simulink library "PB_Library_Master_Working"  (R2021a)
settings: Solver=VariableStepAuto  StartTime=0.0  StopTime=10.0  RelTol=1e-3
undefined symbols (not defined in the file): A_M, B_M, component_degradation_input, E0_M, f_sw, f_sw_M_aDF, flux_m_aDF, Fsw_M_aDF, insert, K_M, L_M_aDF, L_M_adf, P_Fe_Nom_aDF, Q_M, Q_rr, r_c, r_D, R_M, R_s_aDF, resistance_aDF, S_nom_aDF, SOC_Init_M, TFall_M_aDF, TRise_M_aDF, Trr_M_aDF, u_ce0, u_D0
libraries: $bdroot x76, Lib_Dyn_StateSpace_EMTAT x6, Lib_PF_BusLoadDC_TMATS x3, PB_Library_Master x3, simulink x3, TemperatureBlock x1
(part 4 of 5)

== system PB_Library_Master_Working/Rectifier/IGBT Conduction Losses1 ==
  note: You need to read from graphs:
      |
      | -U_ce0
      | -Rc=dU_ce/dI_c (linear)
      | -U_D0
      | -R_D=dU_D/dI_D (linear)
  I_M : Inport
  PF : Inport  Port=2
  m : Inport  Port=3
  T : Inport  Port=4
  1-D Lookup Table r_c : Lookup_n-D  NumberOfTableDimensions=1  BreakpointsForDimension1=T_M  Table=R_c_M  InternalRulePriority=Speed  RndMeth=Simplest  InputSameDT=on
  1-D Lookup Table u_ce0 : Lookup_n-D  NumberOfTableDimensions=1  BreakpointsForDimension1=T_M  Table=u_ce0_M  InternalRulePriority=Speed  RndMeth=Simplest  InputSameDT=on
  Constant : Constant  Value=1/(2*pi)
  Constant1 : Constant  Value=1/8
  Gain : Gain  Commented=on  Gain=u_ce0
  Gain1 : Gain  Gain=1/8
  Gain2 : Gain  Commented=on  Gain=r_c
  Gain3 : Gain  Gain=1/(3*pi)
  Product{,1..4} (5 alike) : Product
  Square : Math  Operator=square  SignedPower=on  SaturateOnIntegerOverflow=on
  Sum : Sum
  Sum2 : Sum
  Sum3 : Sum
  P_CT : Outport  VectorParamsAs1DForOutWhenUnconnected=off
  wires:
  1-D Lookup Table r_c/1 -> Product4/2
  1-D Lookup Table u_ce0/1 -> Product3/2
  T/1 -> 1-D Lookup Table r_c/1, 1-D Lookup Table u_ce0/1
  Sum3/1 -> Product2/2
  Constant1/1 -> Sum3/2
  Product4/1 -> Product2/1
  Gain3/1 -> Sum3/1
  Square/1 -> Product4/1
  Sum/1 -> Product/1
  Product1/1 -> Gain1/1, Gain3/1
  Gain1/1 -> Sum/2
  m/1 -> Product1/2
  PF/1 -> Product1/1
  Constant/1 -> Sum/1
  Product3/1 -> Square/1, Product/2
  I_M/1 -> Product3/1  "I_M"
  Sum2/1 -> P_CT/1
  Product2/1 -> Sum2/2
  Product/1 -> Sum2/1

== system PB_Library_Master_Working/Rectifier/IGBT Switching Losses1 ==
  note: the aDF must increase E1_M
  I_ce : Inport
  T : Inport  Port=2
  1-D Lookup Table E0 : Lookup_n-D  NumberOfTableDimensions=1  BreakpointsForDimension1=T_M  Table=E0_M  InternalRulePriority=Speed  RndMeth=Simplest  InputSameDT=on
  1-D Lookup Table E1 : Lookup_n-D  NumberOfTableDimensions=1  BreakpointsForDimension1=T_M  Table=E1_M  InternalRulePriority=Speed  RndMeth=Simplest  InputSameDT=on
  Add : Sum
  Constant : Constant  Value=f_sw_M
  Constant1 : Constant  Value=[insert f_sw_M_aDF]
  Divide : Product  Inputs=*/
  Product : Product
  Product1 : Product
  P_ST : Outport  VectorParamsAs1DForOutWhenUnconnected=off
  wires:
  Product/1 -> P_ST/1
  Add/1 -> Product/1
  I_ce/1 -> Product1/1
  1-D Lookup Table E0/1 -> Add/1
  Product1/1 -> Add/2
  T/1 -> 1-D Lookup Table E0/1, 1-D Lookup Table E1/1
  1-D Lookup Table E1/1 -> Product1/2
  Constant/1 -> Divide/1
  Divide/1 -> Product/2
  Constant1/1 -> Divide/2

== system PB_Library_Master_Working/Rectifier/I_Ripple1 ==
  V_batt : Inport
  "V_M " : Inport  Port=2
  Constant : Constant  Value=L_s_M
  Constant1 : Constant  Value=[insert f_sw_M_aDF]
  Divide : Product  Inputs=*/
  Divide1 : Product  Inputs=*/
  Gain : Gain  Gain=sqrt(2)
  Gain1 : Gain  Gain=2
  Gain2 : Gain  Gain=f_sw_M
  Product : Product
  Product1 : Product
  Subtract : Sum  Inputs=+-
  I_Rip : Outport  VectorParamsAs1DForOutWhenUnconnected=off
  wires:
  Divide/1 -> I_Rip/1
  Product1/1 -> Gain2/1
  Gain1/1 -> Product1/2
  Constant/1 -> Gain1/1
  Product/1 -> Divide/1
  Subtract/1 -> Product/1
  V_batt/1 -> Product1/1, Subtract/1
  Gain/1 -> Subtract/2
  "V_M "/1 -> Gain/1, Product/2
  Gain2/1 -> Divide1/1
  Constant1/1 -> Divide1/2
  Divide1/1 -> Divide/2

== system PB_Library_Master_Working/Rectifier/P_out_gen ==
  I (RMS) : Inport
  V_s (RMS) : Inport  Port=2
  PF : Inport  Port=3
  Gain : Gain  Gain=sqrt(3)
  Product : Product  Inputs=3
  P_out_gen : Outport  VectorParamsAs1DForOutWhenUnconnected=off
  wires:
  Product/1 -> Gain/1
  Gain/1 -> P_out_gen/1
  V_s (RMS)/1 -> Product/1
  PF/1 -> Product/3
  I (RMS)/1 -> Product/2

== system PB_Library_Master_Working/Rectifier/mVal ==
  V_s : Inport
  V_batt : Inport  Port=2
  Divide : Product  Inputs=*/
  Gain : Gain  Gain=sqrt(2)
  m : Outport  VectorParamsAs1DForOutWhenUnconnected=off
  wires:
  V_batt/1 -> Divide/2
  Gain/1 -> Divide/1
  V_s/1 -> Gain/1
  Divide/1 -> m/1

== system PB_Library_Master_Working/Boost Converter/DC - DC Converter/ Dynamic State ==
  note: On Cycle
  note: Off Cycle
  x : Inport
  u : Inport  Port=2
  d : Inport  Port=3
  Action Port : ActionPort
  Constant : Constant
  Product{,1..3} (4 alike) : Product
  "State Space Model A1, B1, C1, D1" : Lib_Dyn_StateSpace_EMTAT/State Space Model  A_M=[0, 0; 0, -(Ron_M+RL_M)/L_M]  B_M=[0, -1/C_M; 1/L_M, 0]  C_M="[1,  0]"  D_M=[0, RC_M]
  "State Space Model A2, B2, C2, D2" : Subsystem  mask(State Space Model){A_M=[0, 1/C_M; -1/L_M, -(Ron_M+RC_M+RL_M)/L_M], B_M=[0, -1/C_M; 1/L_M, RC_M/L_M], C_M=[1,  RC_M], D_M=[0, -RC_M]}
      mask prompts: A_M "A_M - "A" Matrix"; B_M "B_M - "B" Matrix"; C_M "C_M - "C" Matrix"; D_M "D_M - "D" Matrix"
      mask help:
      | This block represents a state space model that can be placed within an interative subsytem (i.e. the Newton-Raphson solver).
      | The states, x, and inputs, u must be fed into the block. The outputs, y, and state derivatives, x_dot are computed
      | via the standard state space equations. Note that the integrator that computes the states by integrating
      | the state derivatives should be placed outside of the iterative subsystem so that multiple integration steps do not
      | occur per each timestep.
      |
      | Initial conditions must be specified in the integrator blocks, and ABCD matrices specified as block mask parameters.
      mask Display:
      | fprintf('x_dot = Ax+Bu\ny = Cx+Du')
      | port_label('input',1,'x')
      | port_label('input',2,'u')
      | port_label('output',1,'x_dot')
      | port_label('output',2,'y')
  Sum : Sum  Inputs=++|
  Sum1 : Sum  Inputs=++|
  Sum2 : Sum  Inputs=+-
  xdot : Outport  VectorParamsAs1DForOutWhenUnconnected=off
  VB : Outport  Port=2  VectorParamsAs1DForOutWhenUnconnected=off
  wires:
  "State Space Model A1, B1, C1, D1"/1 -> Product/1
  d/1 -> [d]
  Sum2/1 -> Product2/2, Product3/2
  Constant/1 -> Sum2/1
  [x] -> "State Space Model A1, B1, C1, D1"/1
  "State Space Model A1, B1, C1, D1"/2 -> Product1/1
  [u] -> "State Space Model A1, B1, C1, D1"/2
  [d] -> Product1/2, Product/2
  [d] -> Sum2/2
  u/1 -> [u]
  [x] -> "State Space Model A2, B2, C2, D2"/1(x)
  [u] -> "State Space Model A2, B2, C2, D2"/2(u)
  Product3/1 -> Sum1/2
  "State Space Model A2, B2, C2, D2"/2(y) -> Product3/1
  "State Space Model A2, B2, C2, D2"/1(x_dot) -> Product2/1
  Product2/1 -> Sum/2
  x/1 -> [x]
  Product1/1 -> Sum1/1
  Product/1 -> Sum/1
  Sum1/1 -> VB/1  "VB"
  Sum/1 -> xdot/1  "xdot"

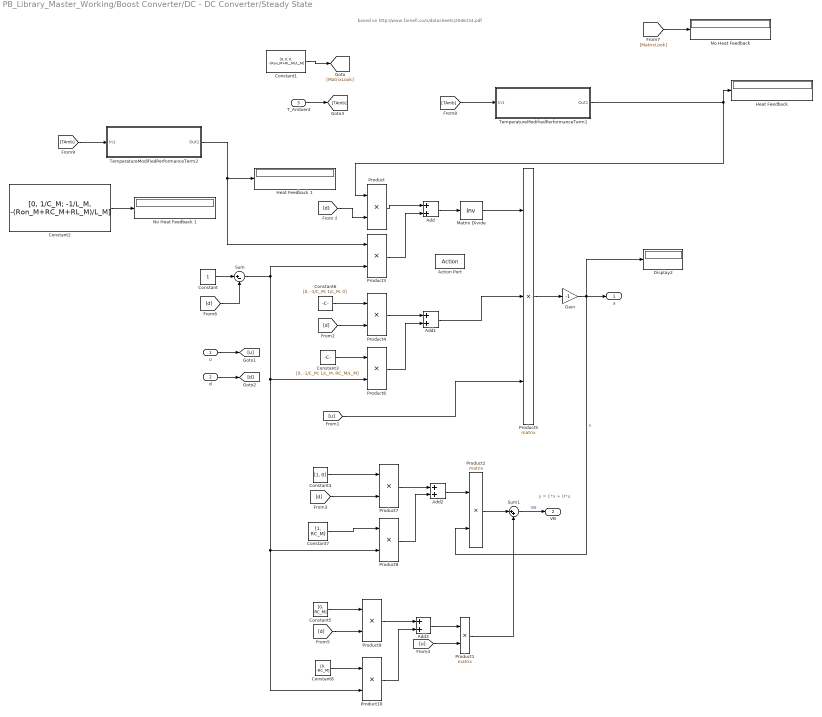
== system PB_Library_Master_Working/Boost Converter/DC - DC Converter/Steady State ==
  note: based on http://www.farnell.com/datasheets/2046154.pdf
  note: d
  note: y = C*x + D*u
  u : Inport
  d : Inport  Port=2
  "T_Ambient " : Inport  Port=3
  Action Port : ActionPort
  Add{,1..3} (4 alike) : Sum
  Constant : Constant
  Constant1 : Constant  Value=[0, 0; 0, -(Ron_M+RL_M)/L_M]  VectorParams1D=off
  Constant2 : Constant  Value=[0, 1/C_M; -1/L_M, -(Ron_M+RC_M+RL_M)/L_M]  VectorParams1D=off
  Constant3 : Constant  Value=[0, -1/C_M; 1/L_M, RC_M/L_M]  VectorParams1D=off
  Constant4 : Constant  Value=[1, 0]  VectorParams1D=off
  Constant5 : Constant  Value=[0, RC_M]  VectorParams1D=off
  Constant6 : Constant  Value=[0, -1/C_M; 1/L_M, 0]  VectorParams1D=off
  Constant7 : Constant  Value=[1, RC_M]  VectorParams1D=off
  Constant8 : Constant  Value=[0, -RC_M]  VectorParams1D=off
  Display2 : Display
  Gain : Gain  Gain=-1
  "Heat Feedback " : Display
  Heat Feedback 1 : Display
  Matrix Divide : Product  Inputs=/  Multiplication=Matrix(*)
  "No Heat Feedback " : Display
  No Heat Feedback 1 : Display
  Product{,3..4,6..10} (8 alike) : Product
  Product1 : Product  Multiplication=Matrix(*)
  Product2 : Product  Multiplication=Matrix(*)
  Product5 : Product  Inputs=3  Multiplication=Matrix(*)
  Sum : Sum  Inputs=|+-
  Sum1 : Sum  Inputs=|++
  "TemperatureModifiedPerformanceTerm1 " : Subsystem
  "TemperatureModifiedPerformanceTerm2 " : Subsystem
  x : Outport  VectorParamsAs1DForOutWhenUnconnected=off
  VB : Outport  Port=2  VectorParamsAs1DForOutWhenUnconnected=off
  wires:
  Constant2/1 -> No Heat Feedback 1/1
  [TAmb] -> "TemperatureModifiedPerformanceTerm2 "/1(In1)
  [TAmb] -> "TemperatureModifiedPerformanceTerm1 "/1(In1)
  "T_Ambient "/1 -> [TAmb]
  "TemperatureModifiedPerformanceTerm2 "/1(Out1) -> Heat Feedback 1/1, Product3/1
  "TemperatureModifiedPerformanceTerm1 "/1(Out1) -> Product/1, "Heat Feedback "/1
  [d] -> Product/2
  [MatrixLook] -> "No Heat Feedback "/1
  Constant8/1 -> Product10/1
  Product6/1 -> Add1/2
  Add/1 -> Matrix Divide/1
  Constant7/1 -> Product8/1
  [d] -> Product7/2
  Add1/1 -> Product5/2
  Product8/1 -> Add2/2
  Product10/1 -> Add3/2
  Constant5/1 -> Product9/1
  [d] -> Sum/2
  Product1/1 -> Sum1/2
  Product5/1 -> Gain/1
  Sum/1 -> Product10/2, Product8/2, Product6/2, Product3/2
  Add3/1 -> Product1/1
  Constant/1 -> Sum/1
  Constant6/1 -> Product4/1
  [u] -> Product5/3
  [d] -> Product4/2
  Gain/1 -> x/1, Display2/1, Product2/2  "x"
  Constant4/1 -> Product7/1
  u/1 -> [u]
  Product2/1 -> Sum1/1
  d/1 -> [d]
  Product7/1 -> Add2/1
  Sum1/1 -> VB/1  "VB"
  Constant1/1 -> [MatrixLook]
  Product4/1 -> Add1/1
  [d] -> Product9/2
  Product/1 -> Add/1
  Constant3/1 -> Product6/1
  Product3/1 -> Add/2
  Matrix Divide/1 -> Product5/1
  Product9/1 -> Add3/1
  Add2/1 -> Product2/1
  [u] -> Product1/2

== system PB_Library_Master_Working/Boost Converter/Power Loss /VGateTempModified ==
  note: normalized to 25°C
  VGate : Inport
  TAmb : Inport  Port=2
  Add1 : Sum
  Constant7 : Constant  Value=25
  Multiply1 : Product
  Subtract : Sum  Inputs=+-
  "V DS temp coefficient " : Constant  Value=.64
  VGateMod : Outport  VectorParamsAs1DForOutWhenUnconnected=off
  wires:
  Add1/1 -> VGateMod/1
  "V DS temp coefficient "/1 -> Multiply1/2
  Subtract/1 -> Multiply1/1
  TAmb/1 -> Subtract/1
  VGate/1 -> Add1/1
  Constant7/1 -> Subtract/2
  Multiply1/1 -> Add1/2

== system PB_Library_Master_Working/Boost Converter Analytic/DC - DC Converter/ Dynamic State ==
  note: On Cycle
  note: Off Cycle
  note: the aDF must decrease L_M
  note: the aDF must decrease L_M
  x : Inport
  u : Inport  Port=2
  d : Inport  Port=3
  Action Port : ActionPort
  Constant : Constant
  Product{,1..3} (4 alike) : Product
  "State Space Model A1, B1, C1, D1" : Lib_Dyn_StateSpace_EMTAT/State Space Model  A_M=[0, 0; 0, -(Ron_M+RL_M)/L_M]  B_M=[0, -1/C_M; 1/L_M, 0]  C_M="[1,  0]"  D_M=[0, RC_M]
  "State Space Model A2, B2, C2, D2" : Subsystem  mask(State Space Model){A_M=[0, 1/C_M; -1/L_M, -(Ron_M+RC_M+RL_M)/L_M], B_M=[0, -1/C_M; 1/L_M, RC_M/L_M], C_M=[1,  RC_M], D_M=[0, -RC_M]}
      mask prompts: A_M "A_M - "A" Matrix"; B_M "B_M - "B" Matrix"; C_M "C_M - "C" Matrix"; D_M "D_M - "D" Matrix"
      mask help:
      | This block represents a state space model that can be placed within an interative subsytem (i.e. the Newton-Raphson solver).
      | The states, x, and inputs, u must be fed into the block. The outputs, y, and state derivatives, x_dot are computed
      | via the standard state space equations. Note that the integrator that computes the states by integrating
      | the state derivatives should be placed outside of the iterative subsystem so that multiple integration steps do not
      | occur per each timestep.
      |
      | Initial conditions must be specified in the integrator blocks, and ABCD matrices specified as block mask parameters.
      mask Display:
      | fprintf('x_dot = Ax+Bu\ny = Cx+Du')
      | port_label('input',1,'x')
      | port_label('input',2,'u')
      | port_label('output',1,'x_dot')
      | port_label('output',2,'y')
  Sum : Sum  Inputs=++|
  Sum1 : Sum  Inputs=++|
  Sum2 : Sum  Inputs=+-
  xdot : Outport  VectorParamsAs1DForOutWhenUnconnected=off
  VB : Outport  Port=2  VectorParamsAs1DForOutWhenUnconnected=off
  wires:
  "State Space Model A1, B1, C1, D1"/1 -> Product/1
  d/1 -> [d]
  Sum2/1 -> Product2/2, Product3/2
  Constant/1 -> Sum2/1
  [x] -> "State Space Model A1, B1, C1, D1"/1
  "State Space Model A1, B1, C1, D1"/2 -> Product1/1
  [u] -> "State Space Model A1, B1, C1, D1"/2
  [d] -> Product1/2, Product/2
  [d] -> Sum2/2
  u/1 -> [u]
  [x] -> "State Space Model A2, B2, C2, D2"/1(x)
  [u] -> "State Space Model A2, B2, C2, D2"/2(u)
  Product3/1 -> Sum1/2
  "State Space Model A2, B2, C2, D2"/2(y) -> Product3/1
  "State Space Model A2, B2, C2, D2"/1(x_dot) -> Product2/1
  Product2/1 -> Sum/2
  x/1 -> [x]
  Product1/1 -> Sum1/1
  Product/1 -> Sum/1
  Sum1/1 -> VB/1  "VB"
  Sum/1 -> xdot/1  "xdot"

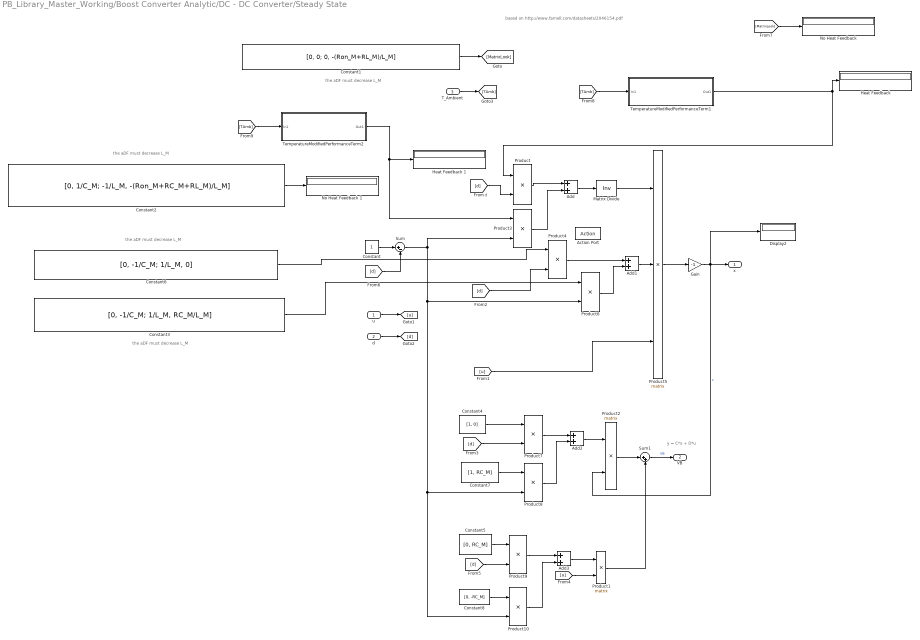
== system PB_Library_Master_Working/Boost Converter Analytic/DC - DC Converter/Steady State ==
  note: the aDF must decrease L_M
  note: based on http://www.farnell.com/datasheets/2046154.pdf
  note: d
  note: y = C*x + D*u
  note: the aDF must decrease L_M
  note: the aDF must decrease L_M
  note: the aDF must decrease L_M
  u : Inport
  d : Inport  Port=2
  "T_Ambient " : Inport  Port=3
  Action Port : ActionPort
  Add{,1..3} (4 alike) : Sum
  Constant : Constant
  Constant1 : Constant  Value=[0, 0; 0, -(Ron_M+RL_M)/L_M]  VectorParams1D=off
  Constant2 : Constant  Value=[0, 1/C_M; -1/L_M, -(Ron_M+RC_M+RL_M)/L_M]  VectorParams1D=off
  Constant3 : Constant  Value=[0, -1/C_M; 1/L_M, RC_M/L_M]  VectorParams1D=off
  Constant4 : Constant  Value=[1, 0]  VectorParams1D=off
  Constant5 : Constant  Value=[0, RC_M]  VectorParams1D=off
  Constant6 : Constant  Value=[0, -1/C_M; 1/L_M, 0]  VectorParams1D=off
  Constant7 : Constant  Value=[1, RC_M]  VectorParams1D=off
  Constant8 : Constant  Value=[0, -RC_M]  VectorParams1D=off
  Display2 : Display
  Gain : Gain  Gain=-1
  "Heat Feedback " : Display
  Heat Feedback 1 : Display
  Matrix Divide : Product  Inputs=/  Multiplication=Matrix(*)
  "No Heat Feedback " : Display
  No Heat Feedback 1 : Display
  Product{,3..4,6..10} (8 alike) : Product
  Product1 : Product  Multiplication=Matrix(*)
  Product2 : Product  Multiplication=Matrix(*)
  Product5 : Product  Inputs=3  Multiplication=Matrix(*)
  Sum : Sum  Inputs=|+-
  Sum1 : Sum  Inputs=|++
  "TemperatureModifiedPerformanceTerm1 " : Subsystem
  "TemperatureModifiedPerformanceTerm2 " : Subsystem
  x : Outport  VectorParamsAs1DForOutWhenUnconnected=off
  VB : Outport  Port=2  VectorParamsAs1DForOutWhenUnconnected=off
  wires:
  Constant2/1 -> No Heat Feedback 1/1
  [TAmb] -> "TemperatureModifiedPerformanceTerm2 "/1(In1)
  [TAmb] -> "TemperatureModifiedPerformanceTerm1 "/1(In1)
  "T_Ambient "/1 -> [TAmb]
  "TemperatureModifiedPerformanceTerm2 "/1(Out1) -> Heat Feedback 1/1, Product3/1
  "TemperatureModifiedPerformanceTerm1 "/1(Out1) -> Product/1, "Heat Feedback "/1
  [d] -> Product/2
  [MatrixLook] -> "No Heat Feedback "/1
  Constant8/1 -> Product10/1
  Product6/1 -> Add1/2
  Add/1 -> Matrix Divide/1
  Constant7/1 -> Product8/1
  [d] -> Product7/2
  Add1/1 -> Product5/2
  Product8/1 -> Add2/2
  Product10/1 -> Add3/2
  Constant5/1 -> Product9/1
  [d] -> Sum/2
  Product1/1 -> Sum1/2
  Product5/1 -> Gain/1
  Sum/1 -> Product10/2, Product8/2, Product6/2, Product3/2
  Add3/1 -> Product1/1
  Constant/1 -> Sum/1
  Constant6/1 -> Product4/1
  [u] -> Product5/3
  [d] -> Product4/2
  Gain/1 -> x/1, Display2/1, Product2/2  "x"
  Constant4/1 -> Product7/1
  u/1 -> [u]
  Product2/1 -> Sum1/1
  d/1 -> [d]
  Product7/1 -> Add2/1
  Sum1/1 -> VB/1  "VB"
  Constant1/1 -> [MatrixLook]
  Product4/1 -> Add1/1
  [d] -> Product9/2
  Product/1 -> Add/1
  Constant3/1 -> Product6/1
  Product3/1 -> Add/2
  Matrix Divide/1 -> Product5/1
  Product9/1 -> Add3/1
  Add2/1 -> Product2/1
  [u] -> Product1/2

== system PB_Library_Master_Working/Boost Converter Analytic/Power Loss /VGateTempModified ==
  note: normalized to 25°C
  VGate : Inport
  TAmb : Inport  Port=2
  Add1 : Sum
  Constant7 : Constant  Value=25
  Multiply1 : Product
  Subtract : Sum  Inputs=+-
  "V DS temp coefficient " : Constant  Value=.64
  VGateMod : Outport  VectorParamsAs1DForOutWhenUnconnected=off
  wires:
  Add1/1 -> VGateMod/1
  "V DS temp coefficient "/1 -> Multiply1/2
  Subtract/1 -> Multiply1/1
  TAmb/1 -> Subtract/1
  VGate/1 -> Add1/1
  Constant7/1 -> Subtract/2
  Multiply1/1 -> Add1/2

== system PB_Library_Master_Working/Buck Converter/DC - DC Converter/ Dynamic State ==
  x : Inport
  u : Inport  Port=2
  d : Inport  Port=3
  Action Port : ActionPort
  Constant : Constant
  Product{,1..3} (4 alike) : Product
  "State Space Model A1, B1, C1, D1" : Lib_Dyn_StateSpace_EMTAT/State Space Model  A_M=[0, 1/C_M; -1/L_M, -(Ron_M+RC_M+RL_M)/L_M]  B_M=[0, -1/C_M; 1/L_M, RC_M/L_M]  C_M="[1,  RC_M]"  D_M=[0, -RC_M]
  "State Space Model A2, B2, C2, D2" : Lib_Dyn_StateSpace_EMTAT/State Space Model  A_M=[0, 1/C_M; -1/L_M, -(Ron_M+RC_M+RL_M)/L_M]  B_M=[0, -1/C_M; 0, RC_M/L_M]  C_M="[1,  RC_M]"  D_M=[0, -RC_M]
  Sum : Sum  Inputs=++|
  Sum1 : Sum  Inputs=++|
  Sum2 : Sum  Inputs=+-
  xdot : Outport  VectorParamsAs1DForOutWhenUnconnected=off
  VB : Outport  Port=2  VectorParamsAs1DForOutWhenUnconnected=off
  wires:
  "State Space Model A1, B1, C1, D1"/1 -> Product/1
  d/1 -> [d]
  Sum2/1 -> Product2/2, Product3/2
  Constant/1 -> Sum2/1
  [x] -> "State Space Model A1, B1, C1, D1"/1
  "State Space Model A1, B1, C1, D1"/2 -> Product1/1
  [u] -> "State Space Model A1, B1, C1, D1"/2
  [d] -> Product1/2, Product/2
  [d] -> Sum2/2
  u/1 -> [u]
  [x] -> "State Space Model A2, B2, C2, D2"/1
  [u] -> "State Space Model A2, B2, C2, D2"/2
  Product3/1 -> Sum1/2
  "State Space Model A2, B2, C2, D2"/2 -> Product3/1
  "State Space Model A2, B2, C2, D2"/1 -> Product2/1
  Product2/1 -> Sum/2
  x/1 -> [x]
  Product1/1 -> Sum1/1
  Product/1 -> Sum/1
  Sum1/1 -> VB/1  "VB"
  Sum/1 -> xdot/1  "xdot"

== system PB_Library_Master_Working/Buck Converter/DC - DC Converter/Steady State ==
  note: d
  note: y = C*x + D*u
  u : Inport
  d : Inport  Port=2
  "T_Ambient " : Inport  Port=3
  Action Port : ActionPort
  Add{,1..3} (4 alike) : Sum
  Constant : Constant
  Constant3 : Constant  Value=[0, -1/C_M; 0, RC_M/L_M]  VectorParams1D=off
  Constant4 : Constant  Value=[1, RC_M]  VectorParams1D=off
  Constant5 : Constant  Value=[0, -RC_M]  VectorParams1D=off
  Constant6 : Constant  Value=[0, -1/C_M; 1/L_M, RC_M]  VectorParams1D=off
  Constant7 : Constant  Value=[1, RC_M]  VectorParams1D=off
  Constant8 : Constant  Value=[0, -RC_M]  VectorParams1D=off
  Gain : Gain  Gain=-1
  Matrix Divide : Product  Inputs=/  Multiplication=Matrix(*)
  Product{,3..4,6..10} (8 alike) : Product
  Product1 : Product  Multiplication=Matrix(*)
  Product2 : Product  Multiplication=Matrix(*)
  Product5 : Product  Inputs=3  Multiplication=Matrix(*)
  Sum : Sum  Inputs=|+-
  Sum1 : Sum  Inputs=|++
  "TemperatureModifiedPerformanceTerm2 " : Subsystem
  x : Outport  VectorParamsAs1DForOutWhenUnconnected=off
  VB : Outport  Port=2  VectorParamsAs1DForOutWhenUnconnected=off
  wires:
  "T_Ambient "/1 -> "TemperatureModifiedPerformanceTerm2 "/1(TAmbient)
  "TemperatureModifiedPerformanceTerm2 "/1(Out1) -> Product3/1, Product/1
  Constant8/1 -> Product10/1
  Product6/1 -> Add1/2
  Add/1 -> Matrix Divide/1
  Constant7/1 -> Product8/1
  [d] -> Product7/2
  Add1/1 -> Product5/2
  Product8/1 -> Add2/2
  Product10/1 -> Add3/2
  [d] -> Product/2
  Constant5/1 -> Product9/1
  [d] -> Sum/2
  Product1/1 -> Sum1/2
  Product5/1 -> Gain/1
  Sum/1 -> Product10/2, Product8/2, Product6/2, Product3/2
  Add3/1 -> Product1/1
  Constant/1 -> Sum/1
  Constant6/1 -> Product4/1
  [u] -> Product5/3
  [d] -> Product4/2
  Gain/1 -> x/1, Product2/2  "x"
  Constant4/1 -> Product7/1
  u/1 -> [u]
  Product2/1 -> Sum1/1
  d/1 -> [d]
  Product7/1 -> Add2/1
  Sum1/1 -> VB/1  "VB"
  Product4/1 -> Add1/1
  [d] -> Product9/2
  Product/1 -> Add/1
  Constant3/1 -> Product6/1
  Product3/1 -> Add/2
  Matrix Divide/1 -> Product5/1
  Product9/1 -> Add3/1
  Add2/1 -> Product2/1
  [u] -> Product1/2

== system PB_Library_Master_Working/Buck Converter/Power Loss /VGateTempModified ==
  note: normalized to 25°C
  "VGate " : Inport
  TAmb : Inport  Port=2
  Add1 : Sum
  Constant7 : Constant  Value=25
  Multiply1 : Product
  Subtract : Sum  Inputs=+-
  "V DS temp coefficient " : Constant  Value=.64
  "VGateMod " : Outport  VectorParamsAs1DForOutWhenUnconnected=off
  wires:
  Add1/1 -> "VGateMod "/1
  "V DS temp coefficient "/1 -> Multiply1/2
  Subtract/1 -> Multiply1/1
  TAmb/1 -> Subtract/1
  "VGate "/1 -> Add1/1
  Constant7/1 -> Subtract/2
  Multiply1/1 -> Add1/2

== system PB_Library_Master_Working/Buck Converter Analytic/DC - DC Converter/ Dynamic State ==
  x : Inport
  u : Inport  Port=2
  d : Inport  Port=3
  Action Port : ActionPort
  Constant : Constant
  Product{,1..3} (4 alike) : Product
  "State Space Model A1, B1, C1, D1" : Lib_Dyn_StateSpace_EMTAT/State Space Model  A_M=[0, 1/C_M; -1/L_M, -(Ron_M+RC_M+RL_M)/L_M]  B_M=[0, -1/C_M; 1/L_M, RC_M/L_M]  C_M="[1,  RC_M]"  D_M=[0, -RC_M]
  "State Space Model A2, B2, C2, D2" : Lib_Dyn_StateSpace_EMTAT/State Space Model  A_M=[0, 1/C_M; -1/L_M, -(Ron_M+RC_M+RL_M)/L_M]  B_M=[0, -1/C_M; 0, RC_M/L_M]  C_M="[1,  RC_M]"  D_M=[0, -RC_M]
  Sum : Sum  Inputs=++|
  Sum1 : Sum  Inputs=++|
  Sum2 : Sum  Inputs=+-
  xdot : Outport  VectorParamsAs1DForOutWhenUnconnected=off
  VB : Outport  Port=2  VectorParamsAs1DForOutWhenUnconnected=off
  wires:
  Sum/1 -> xdot/1  "xdot"
  Sum1/1 -> VB/1  "VB"
  Product/1 -> Sum/1
  Product1/1 -> Sum1/1
  x/1 -> [x]
  Product2/1 -> Sum/2
  "State Space Model A2, B2, C2, D2"/1 -> Product2/1
  "State Space Model A2, B2, C2, D2"/2 -> Product3/1
  Product3/1 -> Sum1/2
  [u] -> "State Space Model A2, B2, C2, D2"/2
  [x] -> "State Space Model A2, B2, C2, D2"/1
  u/1 -> [u]
  [d] -> Sum2/2
  [d] -> Product/2, Product1/2
  [u] -> "State Space Model A1, B1, C1, D1"/2
  "State Space Model A1, B1, C1, D1"/2 -> Product1/1
  [x] -> "State Space Model A1, B1, C1, D1"/1
  Constant/1 -> Sum2/1
  Sum2/1 -> Product3/2, Product2/2
  d/1 -> [d]
  "State Space Model A1, B1, C1, D1"/1 -> Product/1

== system PB_Library_Master_Working/Buck Converter Analytic/DC - DC Converter/Steady State ==
  note: y = C*x + D*u
  note: d
  u : Inport
  d : Inport  Port=2
  "T_Ambient " : Inport  Port=3
  Action Port : ActionPort
  Add{,1..3} (4 alike) : Sum
  Constant : Constant
  Constant3 : Constant  Value=[0, -1/C_M; 0, RC_M/L_M]  VectorParams1D=off
  Constant4 : Constant  Value=[1, RC_M]  VectorParams1D=off
  Constant5 : Constant  Value=[0, -RC_M]  VectorParams1D=off
  Constant6 : Constant  Value=[0, -1/C_M; 1/L_M, RC_M]  VectorParams1D=off
  Constant7 : Constant  Value=[1, RC_M]  VectorParams1D=off
  Constant8 : Constant  Value=[0, -RC_M]  VectorParams1D=off
  Gain : Gain  Gain=-1
  Matrix Divide : Product  Inputs=/  Multiplication=Matrix(*)
  Product{,3..4,6..10} (8 alike) : Product
  Product1 : Product  Multiplication=Matrix(*)
  Product2 : Product  Multiplication=Matrix(*)
  Product5 : Product  Inputs=3  Multiplication=Matrix(*)
  Sum : Sum  Inputs=|+-
  Sum1 : Sum  Inputs=|++
  "TemperatureModifiedPerformanceTerm2 " : Subsystem
  x : Outport  VectorParamsAs1DForOutWhenUnconnected=off
  VB : Outport  Port=2  VectorParamsAs1DForOutWhenUnconnected=off
  wires:
  [u] -> Product1/2
  Add2/1 -> Product2/1
  Product9/1 -> Add3/1
  Matrix Divide/1 -> Product5/1
  Product3/1 -> Add/2
  Constant3/1 -> Product6/1
  Product/1 -> Add/1
  [d] -> Product9/2
  Product4/1 -> Add1/1
  Sum1/1 -> VB/1  "VB"
  Product7/1 -> Add2/1
  d/1 -> [d]
  Product2/1 -> Sum1/1
  u/1 -> [u]
  Constant4/1 -> Product7/1
  Gain/1 -> Product2/2, x/1  "x"
  [d] -> Product4/2
  [u] -> Product5/3
  Constant6/1 -> Product4/1
  Constant/1 -> Sum/1
  Add3/1 -> Product1/1
  Sum/1 -> Product3/2, Product6/2, Product8/2, Product10/2
  Product5/1 -> Gain/1
  Product1/1 -> Sum1/2
  [d] -> Sum/2
  Constant5/1 -> Product9/1
  [d] -> Product/2
  Product10/1 -> Add3/2
  Product8/1 -> Add2/2
  Add1/1 -> Product5/2
  [d] -> Product7/2
  Constant7/1 -> Product8/1
  Add/1 -> Matrix Divide/1
  Product6/1 -> Add1/2
  Constant8/1 -> Product10/1
  "TemperatureModifiedPerformanceTerm2 "/1(Out1) -> Product/1, Product3/1
  "T_Ambient "/1 -> "TemperatureModifiedPerformanceTerm2 "/1(TAmbient)

== system PB_Library_Master_Working/Buck Converter Analytic/Power Loss /VGateTempModified ==
  note: normalized to 25°C
  "VGate " : Inport
  TAmb : Inport  Port=2
  Add1 : Sum
  Constant7 : Constant  Value=25
  Multiply1 : Product
  Subtract : Sum  Inputs=+-
  "V DS temp coefficient " : Constant  Value=.64
  "VGateMod " : Outport  VectorParamsAs1DForOutWhenUnconnected=off
  wires:
  Multiply1/1 -> Add1/2
  Constant7/1 -> Subtract/2
  "VGate "/1 -> Add1/1
  TAmb/1 -> Subtract/1
  Subtract/1 -> Multiply1/1
  "V DS temp coefficient "/1 -> Multiply1/2
  Add1/1 -> "VGateMod "/1

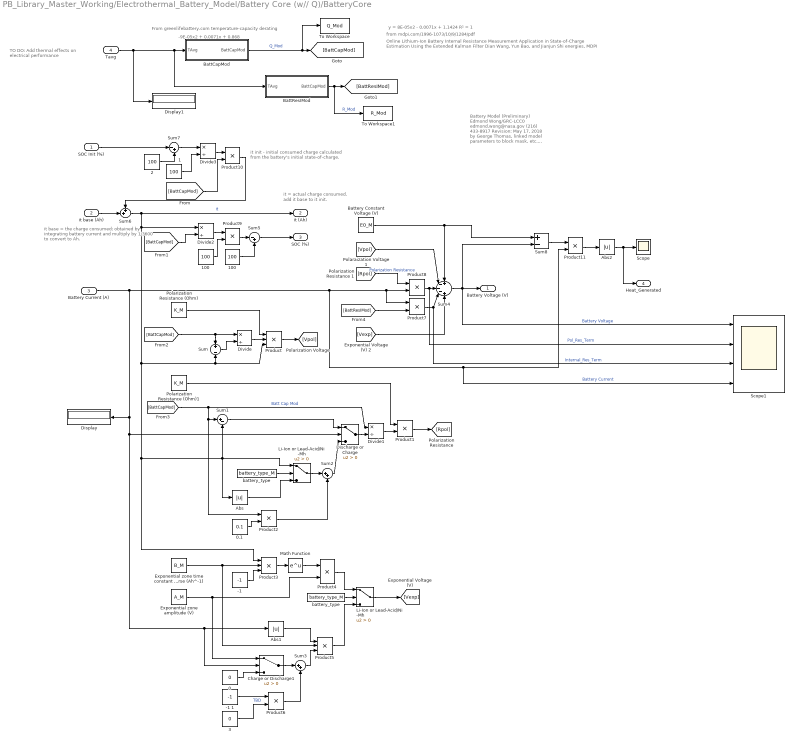
== system PB_Library_Master_Working/Electrothermal_Battery_Model/Battery Core (w// Q)/BatteryCore ==
  note: TO DO: Add thermal effects on electrical performance
  note: it = actual charge consumed.
      | add it base to it init.
  note: it init - initial consumed charge calculated
      | from the battery's initial state-of-charge.
  note: it base = the charge consumed;
      | obtained by integrating battery current
      | and multiply by 1/3600 to convert to Ah.
  note: Battery Model (Preliminary)
      | Edmond Wong/GRC-LCC0
      | edmond.wong@nasa.gov
      | (216) 433-8917
      |
      | Revision: May 17, 2018
      | by George Thomas, linked model
      | parameters to block mask, etc.
      |
      | Revision: April 29, 2019
      | by Mark Bell
      | Heat output, initial temperature feedback
  note: -9E-05x2 + 0.0071x + 0.868
  note: From greenlifebattery.com temperature-capacity derating
  note: y = 8E-05x2 - 0.0071x + 1.1424 R² = 1
  note: from mdpi.com/1996-1073/10/9/1284/pdf
  note: Online Lithium-Ion Battery Internal Resistance Measurement Application in State-of-Charge
      | Estimation Using the Extended Kalman Filter
      |
      | Dian Wang, Yun Bao, and Jianjun Shi
      |
      | energies, MDPI
  "SOC Init (%) " : Inport
  "it base (Ah) " : Inport  Port=2
  "Battery Current (A) " : Inport  Port=3
  "Tavg " : Inport  Port=4
  "-1 " : Constant  Value=-1
  -1 1 : Constant  Value=-1
  0 : Constant  Value=0
  0.1 : Constant  Value=0.1
  1 : Constant  Value=100
  100 : Constant  Value=100
  "100 " : Constant  Value=100
  2 : Constant  Value=100
  3 : Constant  Value=0
  Abs : Abs
  Abs1 : Abs
  Abs2 : Abs
  "BattCapMod " : Subsystem
  "BattResIMod " : Subsystem
  Battery Constant Voltage (V) : Constant  Value=E0_M
  Charge or Discharge1 : Switch  Criteria=u2 > Threshold
  Discharge or Charge : Switch  Criteria=u2 > Threshold
  Display : Display
  Display1 : Display
  Divide{,1..3} (4 alike) : Product  Inputs=*/
  Exponential zone amplitude (V) : Constant  Value=A_M
  Exponential zone time constant inverse (Ah^-1) : Constant  Value=B_M
  Li-Ion or Lead-Acid/Ni-Mh : Switch  Criteria=u2 > Threshold
  "Li-Ion or Lead-Acid/Ni-Mh " : Switch  Criteria=u2 > Threshold
  Math Function : Math  SignedPower=on  SaturateOnIntegerOverflow=on
  Polarization Resistance (Ohm) : Constant  Value=K_M
  Polarization Resistance (Ohm)1 : Constant  Value=K_M
  Product : Product  Inputs=3
  Product{1..2,4,6..11} (9 alike) : Product
  Product3 : Product  Inputs=3
  Product5 : Product  Inputs=3
  Scope : Scope
  Scope1 : Scope  NumInputPorts=4
  Sum : Sum  Inputs=+||-
  Sum1 : Sum  Inputs=|+-
  Sum2 : Sum  Inputs=|++
  Sum3 : Sum  Inputs=|++
  Sum4 : Sum  Inputs=+---+
  Sum5 : Sum  Inputs=|-+
  Sum6 : Sum  Inputs=++|
  Sum7 : Sum  Inputs=|-+
  Sum8 : Sum  Inputs=+-
  To Workspace : ToWorkspace  VariableName=Q_Mod  SampleTime=-1
  To Workspace1 : ToWorkspace  VariableName=R_Mod  SampleTime=-1
  battery_type : Constant  Value=battery_type_M
  "battery_type " : Constant  Value=battery_type_M
  Battery Voltage (V) : Outport  VectorParamsAs1DForOutWhenUnconnected=off
  it (Ah) : Outport  Port=2  VectorParamsAs1DForOutWhenUnconnected=off
  SOC (%) : Outport  Port=3  VectorParamsAs1DForOutWhenUnconnected=off
  Heat_Generated : Outport  Port=4  VectorParamsAs1DForOutWhenUnconnected=off
  wires:
  [BattResIMod] -> Product7/2
  "Tavg "/1 -> Display1/1, "BattCapMod "/1(TAvg), "BattResIMod "/1(TAvg)
  "BattResIMod "/1(BattCapMod) -> To Workspace1/1, [BattResIMod]  "R_Mod"
  [BattCapMod] -> Divide/1, Sum/1
  [BattCapMod] -> Divide2/2
  "BattCapMod "/1(BattCapMod) -> To Workspace/1, [BattCapMod]  "Q_Mod"
  "SOC Init (%) "/1 -> Sum7/1
  Product9/1 -> Sum5/1
  Divide3/1 -> Product10/1
  "100 "/1 -> Sum5/2
  2/1 -> Sum7/2
  Sum7/1 -> Divide3/1
  Product10/1 -> Sum6/1
  "it base (Ah) "/1 -> Sum6/2
  1/1 -> Divide3/2
  Polarization Resistance (Ohm)1/1 -> Product1/1
  Divide/1 -> Product/2
  Product5/1 -> "Li-Ion or Lead-Acid/Ni-Mh "/3
  Product/1 -> [Vpol]
  Sum/1 -> Divide/2
  Product7/1 -> Scope1/3, Sum4/4  "Internal_Res_Term"
  Exponential zone amplitude (V)/1 -> Product4/2, Charge or Discharge1/1
  3/1 -> Product6/2  "TBD"
  Product8/1 -> Scope1/2, Sum4/3  "Pol_Res_Term"
  battery_type/1 -> Li-Ion or Lead-Acid/Ni-Mh/2
  [Vexp] -> Sum4/5
  "battery_type "/1 -> "Li-Ion or Lead-Acid/Ni-Mh "/2
  Product6/1 -> Sum3/2
  Sum6/1 -> Divide2/1, Product/3, Sum/2, Li-Ion or Lead-Acid/Ni-Mh/1, Sum1/2, Abs/1, Product3/1, it (Ah)/1  "it"
  [BattCapMod] -> Divide1/1, Product2/1, Sum1/1  "Batt Cap Mod"
  100/1 -> Product9/2
  "-1 "/1 -> Product3/3
  Charge or Discharge1/1 -> Sum3/1
  Math Function/1 -> Product4/1
  Divide2/1 -> Product9/1
  -1 1/1 -> Product6/1
  [Rpol] -> Product8/1  "Polarization Resistance"
  Sum1/1 -> Discharge or Charge/1
  [Vpol] -> Sum4/2
  Product4/1 -> "Li-Ion or Lead-Acid/Ni-Mh "/1
  Sum5/1 -> SOC (%)/1
  "Li-Ion or Lead-Acid/Ni-Mh "/1 -> [Vexp]
  Polarization Resistance (Ohm)/1 -> Product/1
  Product2/1 -> Sum2/2
  Abs1/1 -> Product5/1
  Discharge or Charge/1 -> Divide1/2
  0/1 -> Charge or Discharge1/3
  Abs/1 -> Li-Ion or Lead-Acid/Ni-Mh/3
  Exponential zone time constant inverse (Ah^-1)/1 -> Product5/2, Product3/2
  Sum2/1 -> Discharge or Charge/3
  Product3/1 -> Math Function/1
  Li-Ion or Lead-Acid/Ni-Mh/1 -> Sum2/1
  Sum3/1 -> Product5/3
  0.1/1 -> Product2/2
  Product1/1 -> [Rpol]
  Divide1/1 -> Product1/2
  Abs2/1 -> Heat_Generated/1, Scope/1
  Sum8/1 -> Product11/1
  Product11/1 -> Abs2/1
  Battery Constant Voltage (V)/1 -> Sum8/1, Sum4/1
  "Battery Current (A) "/1 -> Scope1/4, Product11/2, Product7/1, Product8/2, Discharge or Charge/2, Charge or Discharge1/2, Abs1/1, Display/1  "Battery Current"
  Sum4/1 -> Sum8/2, Battery Voltage (V)/1, Scope1/1  "Battery Voltage"
  [BattCapMod] -> Product10/2

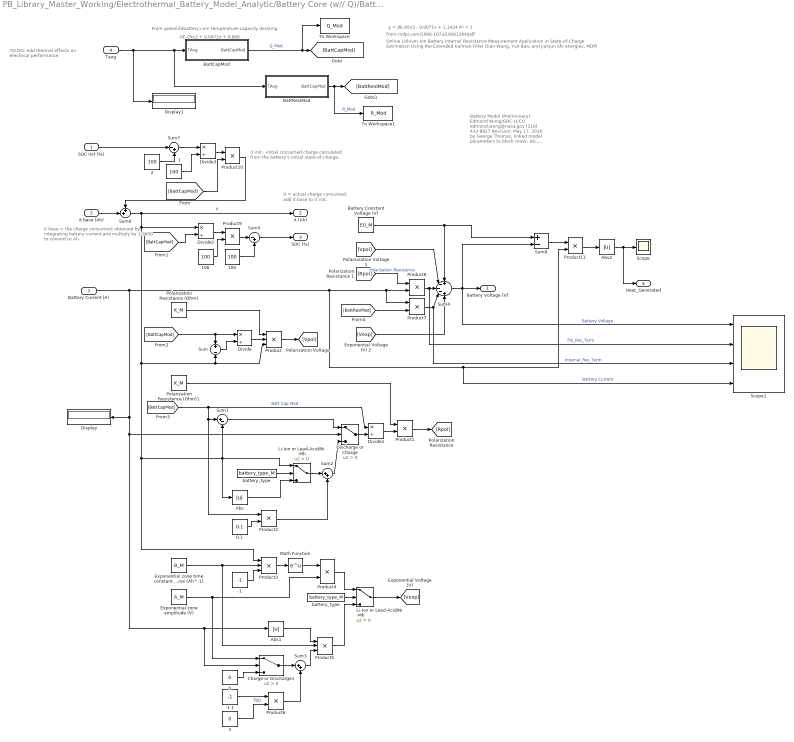
== system PB_Library_Master_Working/Electrothermal_Battery_Model_Analytic/Battery Core (w// Q)/BatteryCore ==
  note: TO DO: Add thermal effects on electrical performance
  note: it = actual charge consumed.
      | add it base to it init.
  note: it init - initial consumed charge calculated
      | from the battery's initial state-of-charge.
  note: it base = the charge consumed;
      | obtained by integrating battery current
      | and multiply by 1/3600 to convert to Ah.
  note: Battery Model (Preliminary)
      | Edmond Wong/GRC-LCC0
      | edmond.wong@nasa.gov
      | (216) 433-8917
      |
      | Revision: May 17, 2018
      | by George Thomas, linked model
      | parameters to block mask, etc.
      |
      | Revision: April 29, 2019
      | by Mark Bell
      | Heat output, initial temperature feedback
  note: -9E-05x2 + 0.0071x + 0.868
  note: From greenlifebattery.com temperature-capacity derating
  note: y = 8E-05x2 - 0.0071x + 1.1424 R² = 1
  note: from mdpi.com/1996-1073/10/9/1284/pdf
  note: Online Lithium-Ion Battery Internal Resistance Measurement Application in State-of-Charge
      | Estimation Using the Extended Kalman Filter
      |
      | Dian Wang, Yun Bao, and Jianjun Shi
      |
      | energies, MDPI
  "SOC Init (%) " : Inport
  "it base (Ah) " : Inport  Port=2
  "Battery Current (A) " : Inport  Port=3
  "Tavg " : Inport  Port=4
  "-1 " : Constant  Value=-1
  -1 1 : Constant  Value=-1
  0 : Constant  Value=0
  0.1 : Constant  Value=0.1
  1 : Constant  Value=100
  100 : Constant  Value=100
  "100 " : Constant  Value=100
  2 : Constant  Value=100
  3 : Constant  Value=0
  Abs : Abs
  Abs1 : Abs
  Abs2 : Abs
  "BattCapMod " : Subsystem
  "BattResIMod " : Subsystem
  Battery Constant Voltage (V) : Constant  Value=E0_M
  Charge or Discharge1 : Switch  Criteria=u2 > Threshold
  Discharge or Charge : Switch  Criteria=u2 > Threshold
  Display : Display
  Display1 : Display
  Divide{,1..3} (4 alike) : Product  Inputs=*/
  Exponential zone amplitude (V) : Constant  Value=A_M
  Exponential zone time constant inverse (Ah^-1) : Constant  Value=B_M
  Li-Ion or Lead-Acid/Ni-Mh : Switch  Criteria=u2 > Threshold
  "Li-Ion or Lead-Acid/Ni-Mh " : Switch  Criteria=u2 > Threshold
  Math Function : Math  SignedPower=on  SaturateOnIntegerOverflow=on
  Polarization Resistance (Ohm) : Constant  Value=K_M
  Polarization Resistance (Ohm)1 : Constant  Value=K_M
  Product : Product  Inputs=3
  Product{1..2,4,6..11} (9 alike) : Product
  Product3 : Product  Inputs=3
  Product5 : Product  Inputs=3
  Scope : Scope
  Scope1 : Scope  NumInputPorts=4
  Sum : Sum  Inputs=+||-
  Sum1 : Sum  Inputs=|+-
  Sum2 : Sum  Inputs=|++
  Sum3 : Sum  Inputs=|++
  Sum4 : Sum  Inputs=+---+
  Sum5 : Sum  Inputs=|-+
  Sum6 : Sum  Inputs=++|
  Sum7 : Sum  Inputs=|-+
  Sum8 : Sum  Inputs=+-
  To Workspace : ToWorkspace  VariableName=Q_Mod  SampleTime=-1
  To Workspace1 : ToWorkspace  VariableName=R_Mod  SampleTime=-1
  battery_type : Constant  Value=battery_type_M
  "battery_type " : Constant  Value=battery_type_M
  Battery Voltage (V) : Outport  VectorParamsAs1DForOutWhenUnconnected=off
  it (Ah) : Outport  Port=2  VectorParamsAs1DForOutWhenUnconnected=off
  SOC (%) : Outport  Port=3  VectorParamsAs1DForOutWhenUnconnected=off
  Heat_Generated : Outport  Port=4  VectorParamsAs1DForOutWhenUnconnected=off
  wires:
  [BattResIMod] -> Product7/2
  "Tavg "/1 -> Display1/1, "BattCapMod "/1(TAvg), "BattResIMod "/1(TAvg)
  "BattResIMod "/1(BattCapMod) -> To Workspace1/1, [BattResIMod]  "R_Mod"
  [BattCapMod] -> Divide/1, Sum/1
  [BattCapMod] -> Divide2/2
  "BattCapMod "/1(BattCapMod) -> To Workspace/1, [BattCapMod]  "Q_Mod"
  "SOC Init (%) "/1 -> Sum7/1
  Product9/1 -> Sum5/1
  Divide3/1 -> Product10/1
  "100 "/1 -> Sum5/2
  2/1 -> Sum7/2
  Sum7/1 -> Divide3/1
  Product10/1 -> Sum6/1
  "it base (Ah) "/1 -> Sum6/2
  1/1 -> Divide3/2
  Polarization Resistance (Ohm)1/1 -> Product1/1
  Divide/1 -> Product/2
  Product5/1 -> "Li-Ion or Lead-Acid/Ni-Mh "/3
  Product/1 -> [Vpol]
  Sum/1 -> Divide/2
  Product7/1 -> Scope1/3, Sum4/4  "Internal_Res_Term"
  Exponential zone amplitude (V)/1 -> Product4/2, Charge or Discharge1/1
  3/1 -> Product6/2  "TBD"
  Product8/1 -> Scope1/2, Sum4/3  "Pol_Res_Term"
  battery_type/1 -> Li-Ion or Lead-Acid/Ni-Mh/2
  [Vexp] -> Sum4/5
  "battery_type "/1 -> "Li-Ion or Lead-Acid/Ni-Mh "/2
  Product6/1 -> Sum3/2
  Sum6/1 -> Divide2/1, Product/3, Sum/2, Li-Ion or Lead-Acid/Ni-Mh/1, Sum1/2, Abs/1, Product3/1, it (Ah)/1  "it"
  [BattCapMod] -> Divide1/1, Product2/1, Sum1/1  "Batt Cap Mod"
  100/1 -> Product9/2
  "-1 "/1 -> Product3/3
  Charge or Discharge1/1 -> Sum3/1
  Math Function/1 -> Product4/1
  Divide2/1 -> Product9/1
  -1 1/1 -> Product6/1
  [Rpol] -> Product8/1  "Polarization Resistance"
  Sum1/1 -> Discharge or Charge/1
  [Vpol] -> Sum4/2
  Product4/1 -> "Li-Ion or Lead-Acid/Ni-Mh "/1
  Sum5/1 -> SOC (%)/1
  "Li-Ion or Lead-Acid/Ni-Mh "/1 -> [Vexp]
  Polarization Resistance (Ohm)/1 -> Product/1
  Product2/1 -> Sum2/2
  Abs1/1 -> Product5/1
  Discharge or Charge/1 -> Divide1/2
  0/1 -> Charge or Discharge1/3
  Abs/1 -> Li-Ion or Lead-Acid/Ni-Mh/3
  Exponential zone time constant inverse (Ah^-1)/1 -> Product5/2, Product3/2
  Sum2/1 -> Discharge or Charge/3
  Product3/1 -> Math Function/1
  Li-Ion or Lead-Acid/Ni-Mh/1 -> Sum2/1
  Sum3/1 -> Product5/3
  0.1/1 -> Product2/2
  Product1/1 -> [Rpol]
  Divide1/1 -> Product1/2
  Abs2/1 -> Heat_Generated/1, Scope/1
  Sum8/1 -> Product11/1
  Product11/1 -> Abs2/1
  Battery Constant Voltage (V)/1 -> Sum8/1, Sum4/1
  "Battery Current (A) "/1 -> Scope1/4, Product11/2, Product7/1, Product8/2, Discharge or Charge/2, Charge or Discharge1/2, Abs1/1, Display/1  "Battery Current"
  Sum4/1 -> Sum8/2, Battery Voltage (V)/1, Scope1/1  "Battery Voltage"
  [BattCapMod] -> Product10/2

== system PB_Library_Master_Working/Boost Converter/DC - DC Converter/ Dynamic State/State Space Model A2, B2, C2, D2 ==
  note: y = C*x + D*u
  note: x_dot = A*x + B*u
  x : Inport
  u : Inport  Port=2
  Constant : Constant  Value=A_M  VectorParams1D=off
  Constant1 : Constant  Value=B_M  VectorParams1D=off
  Constant2 : Constant  Value=C_M  VectorParams1D=off
  Constant3 : Constant  Value=D_M  VectorParams1D=off
  Display{,1..3} (4 alike) : Display
  Product{1..4} (4 alike) : Product  Multiplication=Matrix(*)
  Sum : Sum  Inputs=|++
  Sum1 : Sum  Inputs=|++
  x_dot : Outport  VectorParamsAs1DForOutWhenUnconnected=off
  y : Outport  Port=2  VectorParamsAs1DForOutWhenUnconnected=off
  wires:
  Sum/1 -> x_dot/1, Display2/1
  x/1 -> [x], Display/1
  Sum1/1 -> y/1, Display3/1
  u/1 -> [u], Display1/1
  Constant/1 -> Product4/1
  [x] -> Product4/2
  [u] -> Product3/2
  Constant1/1 -> Product3/1
  Product4/1 -> Sum/1
  Product3/1 -> Sum/2
  Product2/1 -> Sum1/1
  Constant3/1 -> Product1/1
  [x] -> Product2/2
  Product1/1 -> Sum1/2
  [u] -> Product1/2
  Constant2/1 -> Product2/1

== system PB_Library_Master_Working/Boost Converter/DC - DC Converter/Steady State/TemperatureModifiedPerformanceTerm1  ==
  In1 : Inport
  Add5 : Sum
  Constant11 : Constant  Value=-(L_M)
  Constant13 : Constant  Value=0
  Divide1 : Product  Inputs=*/
  "InductorResistance " : Constant  Value=RL_M
  Matrix Concatenate3 : Concatenate  Mode=Multidimensional array
  Matrix Concatenate4 : Concatenate  Mode=Multidimensional array
  Matrix Concatenate5 : Concatenate  Mode=Multidimensional array  ConcatenateDimension=2
  "TModifiedROn " : Subsystem
  Out1 : Outport  VectorParamsAs1DForOutWhenUnconnected=off
  wires:
  Matrix Concatenate5/1 -> Out1/1
  In1/1 -> "TModifiedROn "/1(In1)
  "InductorResistance "/1 -> Add5/1
  "TModifiedROn "/1(Out1) -> Add5/2
  Constant13/1 -> Matrix Concatenate4/1, Matrix Concatenate4/2, Matrix Concatenate3/1
  Matrix Concatenate4/1 -> Matrix Concatenate5/1
  Divide1/1 -> Matrix Concatenate3/2
  Matrix Concatenate3/1 -> Matrix Concatenate5/2
  Add5/1 -> Divide1/1
  Constant11/1 -> Divide1/2

== system PB_Library_Master_Working/Boost Converter/DC - DC Converter/Steady State/TemperatureModifiedPerformanceTerm2  ==
  In1 : Inport
  Add5 : Sum  Inputs=+++
  CapacitorResistance : Constant  Value=RC_M
  Constant : Constant  Value=-1/L_M
  Constant1 : Constant  Value=1/C_M
  Constant11 : Constant  Value=-(L_M)
  Constant13 : Constant  Value=0
  Divide1 : Product  Inputs=*/
  "InductorResistance " : Constant  Value=RL_M
  Matrix Concatenate3 : Concatenate  Mode=Multidimensional array
  Matrix Concatenate4 : Concatenate  Mode=Multidimensional array
  Matrix Concatenate5 : Concatenate  Mode=Multidimensional array  ConcatenateDimension=2
  "TModifiedROn " : Subsystem
  Out1 : Outport  VectorParamsAs1DForOutWhenUnconnected=off
  wires:
  Constant/1 -> Matrix Concatenate4/2
  Constant1/1 -> Matrix Concatenate3/1
  CapacitorResistance/1 -> Add5/3
  Matrix Concatenate5/1 -> Out1/1
  In1/1 -> "TModifiedROn "/1(In1)
  "InductorResistance "/1 -> Add5/1
  "TModifiedROn "/1(Out1) -> Add5/2
  Constant13/1 -> Matrix Concatenate4/1
  Matrix Concatenate4/1 -> Matrix Concatenate5/1
  Divide1/1 -> Matrix Concatenate3/2
  Matrix Concatenate3/1 -> Matrix Concatenate5/2
  Add5/1 -> Divide1/1
  Constant11/1 -> Divide1/2

== system PB_Library_Master_Working/Boost Converter Analytic/DC - DC Converter/ Dynamic State/State Space Model A2, B2, C2, D2 ==
  note: y = C*x + D*u
  note: x_dot = A*x + B*u
  x : Inport
  u : Inport  Port=2
  Constant : Constant  Value=A_M  VectorParams1D=off
  Constant1 : Constant  Value=B_M  VectorParams1D=off
  Constant2 : Constant  Value=C_M  VectorParams1D=off
  Constant3 : Constant  Value=D_M  VectorParams1D=off
  Display{,1..3} (4 alike) : Display
  Product{1..4} (4 alike) : Product  Multiplication=Matrix(*)
  Sum : Sum  Inputs=|++
  Sum1 : Sum  Inputs=|++
  x_dot : Outport  VectorParamsAs1DForOutWhenUnconnected=off
  y : Outport  Port=2  VectorParamsAs1DForOutWhenUnconnected=off
  wires:
  Sum/1 -> x_dot/1, Display2/1
  x/1 -> [x], Display/1
  Sum1/1 -> y/1, Display3/1
  u/1 -> [u], Display1/1
  Constant/1 -> Product4/1
  [x] -> Product4/2
  [u] -> Product3/2
  Constant1/1 -> Product3/1
  Product4/1 -> Sum/1
  Product3/1 -> Sum/2
  Product2/1 -> Sum1/1
  Constant3/1 -> Product1/1
  [x] -> Product2/2
  Product1/1 -> Sum1/2
  [u] -> Product1/2
  Constant2/1 -> Product2/1

== system PB_Library_Master_Working/Boost Converter Analytic/DC - DC Converter/Steady State/TemperatureModifiedPerformanceTerm1  ==
  In1 : Inport
  Add5 : Sum
  Constant : Constant  Value=[insert L_M_aDF]
  Constant11 : Constant  Value=-(L_M)
  Constant13 : Constant  Value=0
  Divide1 : Product  Inputs=*/
  "InductorResistance " : Constant  Value=RL_M
  Matrix Concatenate3 : Concatenate  Mode=Multidimensional array
  Matrix Concatenate4 : Concatenate  Mode=Multidimensional array
  Matrix Concatenate5 : Concatenate  Mode=Multidimensional array  ConcatenateDimension=2
  Product : Product
  "TModifiedROn " : Subsystem
  Out1 : Outport  VectorParamsAs1DForOutWhenUnconnected=off
  wires:
  Matrix Concatenate5/1 -> Out1/1
  In1/1 -> "TModifiedROn "/1(In1)
  "InductorResistance "/1 -> Add5/1
  "TModifiedROn "/1(Out1) -> Add5/2
  Constant13/1 -> Matrix Concatenate4/1, Matrix Concatenate4/2, Matrix Concatenate3/1
  Matrix Concatenate4/1 -> Matrix Concatenate5/1
  Divide1/1 -> Matrix Concatenate3/2
  Matrix Concatenate3/1 -> Matrix Concatenate5/2
  Add5/1 -> Divide1/1
  Product/1 -> Divide1/2
  Constant11/1 -> Product/1
  Constant/1 -> Product/2

== system PB_Library_Master_Working/Boost Converter Analytic/DC - DC Converter/Steady State/TemperatureModifiedPerformanceTerm2  ==
  In1 : Inport
  Add5 : Sum  Inputs=+++
  CapacitorResistance : Constant  Value=RC_M
  Constant : Constant  Value=-1/L_M
  Constant1 : Constant  Value=1/C_M
  Constant11 : Constant  Value=-(L_M)
  Constant13 : Constant  Value=0
  Constant2 : Constant  Value=[insert L_M_adf]
  Constant3 : Constant  Value=[insert L_M_adf]
  Divide : Product  Inputs=*/
  Divide1 : Product  Inputs=*/
  "InductorResistance " : Constant  Value=RL_M
  Matrix Concatenate3 : Concatenate  Mode=Multidimensional array
  Matrix Concatenate4 : Concatenate  Mode=Multidimensional array
  Matrix Concatenate5 : Concatenate  Mode=Multidimensional array  ConcatenateDimension=2
  Product : Product
  "TModifiedROn " : Subsystem
  Out1 : Outport  VectorParamsAs1DForOutWhenUnconnected=off
  wires:
  Constant1/1 -> Matrix Concatenate3/1
  CapacitorResistance/1 -> Add5/3
  Matrix Concatenate5/1 -> Out1/1
  In1/1 -> "TModifiedROn "/1(In1)
  "InductorResistance "/1 -> Add5/1
  "TModifiedROn "/1(Out1) -> Add5/2
  Constant13/1 -> Matrix Concatenate4/1
  Matrix Concatenate4/1 -> Matrix Concatenate5/1
  Divide1/1 -> Matrix Concatenate3/2
  Matrix Concatenate3/1 -> Matrix Concatenate5/2
  Add5/1 -> Divide1/1
  Divide/1 -> Matrix Concatenate4/2
  Constant/1 -> Divide/1
  Constant2/1 -> Divide/2
  Product/1 -> Divide1/2
  Constant11/1 -> Product/1
  Constant3/1 -> Product/2

== system PB_Library_Master_Working/Buck Converter/DC - DC Converter/Steady State/TemperatureModifiedPerformanceTerm2  ==
  TAmbient : Inport
  Add5 : Sum  Inputs=+++
  CapacitorResistance : Constant  Value=RC_M
  Constant : Constant  Value=-1/L_M
  Constant1 : Constant  Value=1/C_M
  Constant11 : Constant  Value=-(L_M)
  Constant13 : Constant  Value=0
  Divide1 : Product  Inputs=*/
  "InductorResistance " : Constant  Value=RL_M
  Matrix Concatenate3 : Concatenate  Mode=Multidimensional array
  Matrix Concatenate4 : Concatenate  Mode=Multidimensional array
  Matrix Concatenate5 : Concatenate  Mode=Multidimensional array  ConcatenateDimension=2
  "TModifiedROn " : Subsystem
  Out1 : Outport  VectorParamsAs1DForOutWhenUnconnected=off
  wires:
  Constant/1 -> Matrix Concatenate4/2
  Constant1/1 -> Matrix Concatenate3/1
  CapacitorResistance/1 -> Add5/3
  Matrix Concatenate5/1 -> Out1/1
  TAmbient/1 -> "TModifiedROn "/1(In1)
  "InductorResistance "/1 -> Add5/1
  "TModifiedROn "/1(Out1) -> Add5/2
  Constant13/1 -> Matrix Concatenate4/1
  Matrix Concatenate4/1 -> Matrix Concatenate5/1
  Divide1/1 -> Matrix Concatenate3/2
  Matrix Concatenate3/1 -> Matrix Concatenate5/2
  Add5/1 -> Divide1/1
  Constant11/1 -> Divide1/2

== system PB_Library_Master_Working/Buck Converter Analytic/DC - DC Converter/Steady State/TemperatureModifiedPerformanceTerm2  ==
  TAmbient : Inport
  Add5 : Sum  Inputs=+++
  CapacitorResistance : Constant  Value=RC_M
  Constant : Constant  Value=-1/L_M
  Constant1 : Constant  Value=1/C_M
  Constant11 : Constant  Value=-(L_M)
  Constant13 : Constant  Value=0
  Divide1 : Product  Inputs=*/
  "InductorResistance " : Constant  Value=RL_M
  Matrix Concatenate3 : Concatenate  Mode=Multidimensional array
  Matrix Concatenate4 : Concatenate  Mode=Multidimensional array
  Matrix Concatenate5 : Concatenate  Mode=Multidimensional array  ConcatenateDimension=2
  "TModifiedROn " : Subsystem
  Out1 : Outport  VectorParamsAs1DForOutWhenUnconnected=off
  wires:
  Constant11/1 -> Divide1/2
  Add5/1 -> Divide1/1
  Matrix Concatenate3/1 -> Matrix Concatenate5/2
  Divide1/1 -> Matrix Concatenate3/2
  Matrix Concatenate4/1 -> Matrix Concatenate5/1
  Constant13/1 -> Matrix Concatenate4/1
  "TModifiedROn "/1(Out1) -> Add5/2
  "InductorResistance "/1 -> Add5/1
  TAmbient/1 -> "TModifiedROn "/1(In1)
  Matrix Concatenate5/1 -> Out1/1
  CapacitorResistance/1 -> Add5/3
  Constant1/1 -> Matrix Concatenate3/1
  Constant/1 -> Matrix Concatenate4/2

== system PB_Library_Master_Working/Electrothermal_Battery_Model/Battery Core (w// Q)/BatteryCore/BattCapMod  ==
  TAvg : Inport
  "A " : Constant  Value=-9e-05
  Add : Sum  Inputs=+++
  "B " : Constant  Value=0.0071
  Battery Capacity (Ah) : Constant  Value=Q_M
  C : Constant  Value=.868
  Multiply : Product
  Multiply1 : Product
  Multiply2 : Product
  Square : Math  Operator=square  SignedPower=on  SaturateOnIntegerOverflow=on
  BattCapMod : Outport  VectorParamsAs1DForOutWhenUnconnected=off
  wires:
  Multiply2/1 -> BattCapMod/1
  C/1 -> Add/3
  Multiply1/1 -> Add/2
  Add/1 -> Multiply2/2
  "A "/1 -> Multiply/2
  Multiply/1 -> Add/1
  Square/1 -> Multiply/1
  TAvg/1 -> Square/1, Multiply1/1
  Battery Capacity (Ah)/1 -> Multiply2/1
  "B "/1 -> Multiply1/2

== system PB_Library_Master_Working/Electrothermal_Battery_Model/Battery Core (w// Q)/BatteryCore/BattResIMod  ==
  TAvg : Inport
  "A " : Constant  Value=8e-05
  Add : Sum  Inputs=+++
  "B " : Constant  Value=0.0071
  C : Constant  Value=1.1424
  Internal Resistance (Ohm) : Constant  Value=R_M
  Multiply : Product
  Multiply1 : Product
  Multiply2 : Product
  Square : Math  Operator=square  SignedPower=on  SaturateOnIntegerOverflow=on
  BattCapMod : Outport  VectorParamsAs1DForOutWhenUnconnected=off
  wires:
  Multiply2/1 -> BattCapMod/1
  C/1 -> Add/3
  Multiply1/1 -> Add/2
  Add/1 -> Multiply2/2
  "A "/1 -> Multiply/2
  Multiply/1 -> Add/1
  Square/1 -> Multiply/1
  TAvg/1 -> Square/1, Multiply1/1
  Internal Resistance (Ohm)/1 -> Multiply2/1
  "B "/1 -> Multiply1/2

== system PB_Library_Master_Working/Electrothermal_Battery_Model_Analytic/Battery Core (w// Q)/BatteryCore/BattCapMod  ==
  TAvg : Inport
  "A " : Constant  Value=-9e-05
  Add : Sum  Inputs=+++
  "B " : Constant  Value=0.0071
  Battery Capacity (Ah) : Constant  Value=Q_M
  C : Constant  Value=.868
  Constant : Constant
  Degradation Parameter Multiplier : $bdroot/Degradation Parameter Multiplier  SystemSampleTime=-1  VariantActivationTime=update diagram  Latency=0  AutoFrameSizeCalculation=off
  Multiply{,1..3} (4 alike) : Product
  Square : Math  Operator=square  SignedPower=on  SaturateOnIntegerOverflow=on
  BattCapMod : Outport  VectorParamsAs1DForOutWhenUnconnected=off
  wires:
  Multiply2/1 -> BattCapMod/1
  C/1 -> Add/3
  Multiply1/1 -> Add/2
  Add/1 -> Multiply2/2
  "A "/1 -> Multiply/2
  Multiply/1 -> Add/1
  Square/1 -> Multiply/1
  TAvg/1 -> Square/1, Multiply1/1
  "B "/1 -> Multiply1/2
  Constant/1 -> Degradation Parameter Multiplier/1
  Battery Capacity (Ah)/1 -> Multiply3/2
  Degradation Parameter Multiplier/1 -> Multiply3/1
  Multiply3/1 -> Multiply2/1

== system PB_Library_Master_Working/Electrothermal_Battery_Model_Analytic/Battery Core (w// Q)/BatteryCore/BattResIMod  ==
  TAvg : Inport
  "A " : Constant  Value=8e-05
  Add : Sum  Inputs=+++
  "B " : Constant  Value=0.0071
  C : Constant  Value=1.1424
  Constant : Constant  Commented=on
  Degradation Parameter Multiplier : $bdroot/Degradation Parameter Multiplier  Commented=on  SystemSampleTime=-1  VariantActivationTime=update diagram  Latency=0  AutoFrameSizeCalculation=off
  Divide : Product  Commented=on  Inputs=/*
  Internal Resistance (Ohm) : Constant  Value=R_M
  Multiply : Product
  Multiply1 : Product
  Multiply2 : Product  Inputs=3
  Square : Math  Operator=square  SignedPower=on  SaturateOnIntegerOverflow=on
  BattCapMod : Outport  VectorParamsAs1DForOutWhenUnconnected=off
  wires:
  Multiply2/1 -> BattCapMod/1
  C/1 -> Add/3
  Multiply1/1 -> Add/2
  Add/1 -> Multiply2/3
  "A "/1 -> Multiply/2
  Multiply/1 -> Add/1
  Square/1 -> Multiply/1
  TAvg/1 -> Square/1, Multiply1/1
  "B "/1 -> Multiply1/2
  Divide/1 -> Multiply2/2
  Degradation Parameter Multiplier/1 -> Divide/1
  Internal Resistance (Ohm)/1 -> Multiply2/1
  Constant/1 -> Degradation Parameter Multiplier/1
